simulink model "PWM2"  (Simulink 7.4)
settings: Solver=ode1  SolverMode=SingleTasking  StartTime=0.0  StopTime=inf  FixedStep=0.01  MaxStep=0.02  RelTol=1e-3  AbsTol=1e-6
CloseFcn:
  | rtwprivate ssgencode ModelCloseRequest MC_AD
settings Model: Creator=Admin  LastModifiedBy=fw  SimulationMode=external  ExtModeTrigDuration=10000
settings ConfigSet: Description=rtmc9s12target_R2009b
settings DataIOCC: LimitDataPoints=off  SaveOutput=off  SaveTime=off  SignalLoggingName=sigsOut
settings OptimizationCC: BlockReduction=off  BooleanDataType=off  InitFltsAndDblsToZero=on  OptimizeModelRefInitCode=on  LifeSpan=1
settings DebuggingCC: SaveWithParameterizedLinksMsg=none  SignalResolutionControl=TryResolveAllWithWarning  SolverPrmCheckMsg=none  MultiTaskDSMMsg=warning  MultiTaskCondExecSysMsg=none  StrictBusMsg=None
settings HardwareCC: ProdBitPerInt=16  ProdEndianess=BigEndian  ProdWordSize=16  ProdHWDeviceType=Motorola HC12
settings RTWCC: SystemTargetFile=mc9s12.tlc  GenerateMakefile=off  TemplateMakefile=mc9s12.tmf  ProcessScript=mc9s12_make_rtw_hook  IncludeERTFirstTime=on
settings CodeAppCC: IgnoreCustomStorageClasses=off
settings STFCustomTargetCC: TargetFcnLib=ansi_tfl_tmw.mat  ModelReferenceCompliant=off  IncludeMdlTerminateFcn=off  ERTCustomFileBanners=on  SupportNonInlinedSFcns=off  CPPClassGenCompliant=on  SystemTargetFile=mc9s12.tlc
settings ERTTargetCC: TargetFcnLib=ansi_tfl_tmw.mat  MultiwordLength=2048  ModelReferenceCompliant=off  ParMdlRefBuildCompliant=off  CompOptLevelCompliant=off  IncludeMdlTerminateFcn=off  CombineOutputUpdateFcns=off  ERTFirstTimeCompliant=off  SupportContinuousTime=on  ModelStepFunctionPrototypeControlCompliant=off  ExtMode=on  ExtModeMexFile=ext_serial_mc9s12_comm  ExtModeMexArgs=1,2,115200  InlinedParameterPlacement=NonHierarchical  ERTCustomFileTemplate=mc9s12_file_process.tlc  GRTInterface=on  ConvertIfToSwitch=off
settings CustomProperty: DataType=RTWOptions_EnumType_C__Users_fw__SVN_rtmc9s12-target_trunk_rtmc9s12_CW_R2009b_bin_mc9s12_1mc9s12_TargetBoard  Value=Dragon12Plus
settings EnumStrPairs: String=Dragon12

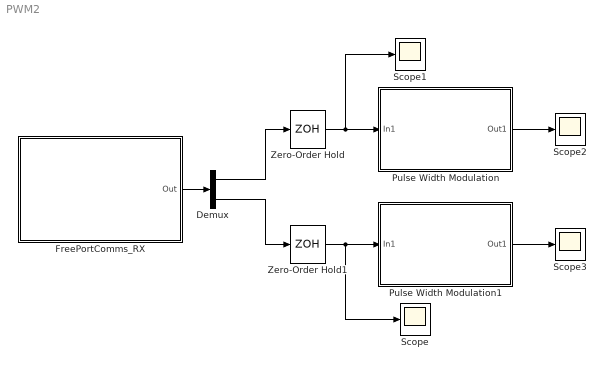
== system PWM2 ==
  Demux : Demux  Outputs=2
  FreePortComms_RX : Subsystem  Tag=mcTarget_freePortCommsRX  mask{sampletime=0.1, port=SCI0, baudrate=115200, channel=0, buf_size=2, data_type=SINGLE, format=off, outformat=on}
      mask prompts: sampletime "Sample time"; port "Communication port"; channel "Channel number"; buf_size "Number of elements"; data_type "Data Type"; format "Block receives raw data"; outformat "Block output is double"
      mask init:
      | [buf_sizestr, portNamestr, baudratestr, channelstr, data_type_str, sampletime_str] = mbc_freeportrxd(sampletime, port, baudrate, channel, buf_size, data_type, format, outformat);
      mask Help: web('freePortComms_rxd.html');
      mask StyleString: edit,popup(SCI0|SCI1|COM1|COM2|COM3|COM4),popup(300|600|1200|2400|4800|9600|19200|38400|57600|115200),edit,edit,popup(SINGLE|INT8|UINT8|INT16|UINT16|INT32|UINT32|BOOLEAN),checkbox,checkbox
      mask Display: fprintf('Receive %s element(s)\nComm port: %s\nBaudrate: %s bps\nChannel: %s\nData type: %s\n Sample rate: %s', buf_sizestr, portNamestr, baudratestr, channelstr, data_type_str, sampletime_str)
  Pulse Width Modulation : Subsystem  Tag=mcTarget_pwm  mask{sampletime=0.01, resolution=16 bit, PWMperiod=0.5, pulse_pin=1  (8-bit / 16-bit), sign_port=PTH, sign_pin=1, Vmax=5, sig_mon=on}
      mask prompts: sampletime "Sample time"; PWMperiod "PWM period (8-bit : up to 0.699 s, 16-bit : up to 179 s)"; pulse_pin "Pulse pin (PTP)"; sign_port "Sign port"; sign_pin "Sign pin"; Vmax "Saturation input level [simulated voltage]"; sig_mon "Signal monitoring"
      mask init:
      | [pulsepinstr, signportstr, signpinstr, periodstr, clkABstr, resstr] = mbc_pwmoutput(sampletime, resolution, PWMperiod, pulse_pin, sign_port, sign_pin, Vmax, sig_mon);
      mask Help: web('pwm_sfcn_9S12.html');
      mask StyleString: edit,popup(8 bit|16 bit),edit,popup(0  (8-bit)|1  (8-bit / 16-bit)|2  (8-bit)|3  (8-bit / 16-bit)|4  (8-bit)|5  (8-bit / 16-bit)|6  (8-bit)|7  (8-bit / 16-bit)),popup(PORTA|PORTB|PTH|PTJ|PTM|PTP|PTT|PTS),popup(0|1|2|3|4|5|6|7),edit,checkbox
      mask Display: fprintf('PWM-%s, %s-bit\nPulse pin: PTP.%s\nSign pin: %s.%s\nPeriod: %s (s)\nSaturation: %d', clkABstr, resstr, pulsepinstr, signportstr, signpinstr, periodstr, Vmax)
  Pulse Width Modulation1 : Subsystem  Tag=mcTarget_pwm  mask{sampletime=0.01, resolution=16 bit, PWMperiod=0.5, pulse_pin=3  (8-bit / 16-bit), sign_port=PTH, sign_pin=2, Vmax=5, sig_mon=on}
      mask prompts: sampletime "Sample time"; PWMperiod "PWM period (8-bit : up to 0.699 s, 16-bit : up to 179 s)"; pulse_pin "Pulse pin (PTP)"; sign_port "Sign port"; sign_pin "Sign pin"; Vmax "Saturation input level [simulated voltage]"; sig_mon "Signal monitoring"
      mask init:
      | [pulsepinstr, signportstr, signpinstr, periodstr, clkABstr, resstr] = mbc_pwmoutput(sampletime, resolution, PWMperiod, pulse_pin, sign_port, sign_pin, Vmax, sig_mon);
      mask Help: web('pwm_sfcn_9S12.html');
      mask StyleString: edit,popup(8 bit|16 bit),edit,popup(0  (8-bit)|1  (8-bit / 16-bit)|2  (8-bit)|3  (8-bit / 16-bit)|4  (8-bit)|5  (8-bit / 16-bit)|6  (8-bit)|7  (8-bit / 16-bit)),popup(PORTA|PORTB|PTH|PTJ|PTM|PTP|PTT|PTS),popup(0|1|2|3|4|5|6|7),edit,checkbox
      mask Display: fprintf('PWM-%s, %s-bit\nPulse pin: PTP.%s\nSign pin: %s.%s\nPeriod: %s (s)\nSaturation: %d', clkABstr, resstr, pulsepinstr, signportstr, signpinstr, periodstr, Vmax)
  Scope{,1..3} (4 alike) : Scope
      Scope settings: TimeRange=10  YMin=-6  YMax=6
      Scope1 settings: TimeRange=10  YMin=-6  YMax=6
      Scope2 settings: TimeRange=0.5  YMin=-6  YMax=6  SaveName=ScopeData2
      Scope3 settings: TimeRange=0.5  YMin=-6  YMax=6  SaveName=ScopeData3
  Zero-Order Hold : ZeroOrderHold  SampleTime=0.01
  Zero-Order Hold1 : ZeroOrderHold  SampleTime=0.01
  wires:
  Zero-Order Hold/1 -> Scope1/1, Pulse Width Modulation/1(In1)
  Zero-Order Hold1/1 -> Scope/1, Pulse Width Modulation1/1(In1)
  FreePortComms_RX/1(Out) -> Demux/1
  Demux/1 -> Zero-Order Hold/1
  Demux/2 -> Zero-Order Hold1/1
  Pulse Width Modulation1/1(Out1) -> Scope3/1
  Pulse Width Modulation/1(Out1) -> Scope2/1

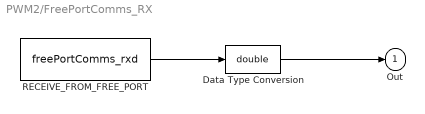
== system PWM2/FreePortComms_RX ==
  Data Type Conversion : DataTypeConversion  OutDataTypeMode=double  OutDataType=sfix(16)  OutScaling=2^0  OutDataTypeStr=double  SaturateOnIntegerOverflow=on  RndMeth=Zero
  RECEIVE_FROM_FREE_PORT : S-Function  Tag=mcTarget_freePortCommsRX  FunctionName=freePortComms_rxd  Parameters=sampletime, channel, buf_size, data_type, port, baudrate, format  EnableBusSupport=off
  Out : Outport  OutDataType=sfix(16)  OutScaling=2^0
  wires:
  RECEIVE_FROM_FREE_PORT/1 -> Data Type Conversion/1
  Data Type Conversion/1 -> Out/1

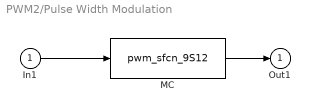
== system PWM2/Pulse Width Modulation ==
  In1 : Inport  OutDataType=sfix(16)  OutScaling=2^0
  MC : S-Function  Tag=mcTarget_pwm  FunctionName=pwm_sfcn_9S12  Parameters=sampletime, PWMperiod, pulse_pin, sign_port, sign_pin, Vmax, sig_mon  EnableBusSupport=off
  Out1 : Outport
  wires:
  In1/1 -> MC/1
  MC/1 -> Out1/1

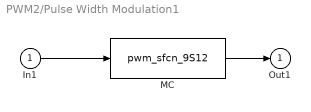
== system PWM2/Pulse Width Modulation1 ==
  In1 : Inport  OutDataType=sfix(16)  OutScaling=2^0
  MC : S-Function  Tag=mcTarget_pwm  FunctionName=pwm_sfcn_9S12  Parameters=sampletime, PWMperiod, pulse_pin, sign_port, sign_pin, Vmax, sig_mon  EnableBusSupport=off
  Out1 : Outport
  wires:
  MC/1 -> Out1/1
  In1/1 -> MC/1
